simulink model "shield_test_model"  (R2024b)
settings: Solver=FixedStepDiscrete  StartTime=0.0  StopTime=5  FixedStep=1  RelTol=1e-3
libraries: simulink x1
settings Model: Creator=luiz-villa  LastModifiedBy=luiz-villa

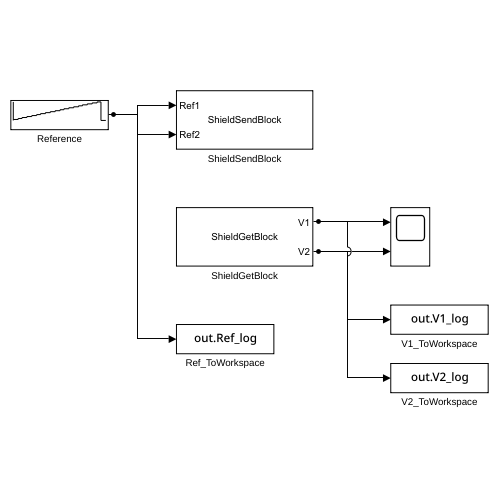
[thumbnail: Simulink's stored preview of the top-level diagram]
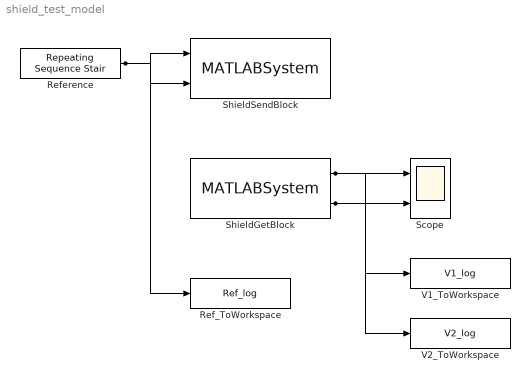
== system shield_test_model ==
  Ref_ToWorkspace : ToWorkspace  VariableName=Ref_log  SampleTime=-1
  Reference : simulink/Sources/Repeating Sequence Stair  OutValues=[5.5 6 6.5 7 7.5 8 8.5 9 9.5 10 10.5 11 11.5 12 12.5 13 13.5 14 14.5 5]  tsamp=1  OutMin=[]  OutMax=[]  OutDataTypeStr=double  OutputDataTypeScalingMode=double  OutDataType=fixdt(0,8)  ConRadixGroup=Best Precision: Vector-wise  OutScaling=2^-12
  Scope : Scope  NumInputPorts=2
  ShieldGetBlock : MATLABSystem  System=ShieldGetBlock  SampleTime=1  VendorID=2fe3  ProductID=0101  Interactive=off
      mask Type: ShieldGetBlock
      mask Display:
      | disp('ShieldGetBlock');
      | port_label('output',1,'V1');
      | port_label('output',2,'V2');
  ShieldSendBlock : MATLABSystem  System=ShieldSendBlock  SampleTime=1  VendorID=2fe3  ProductID=0101  Interactive=off
      mask Type: ShieldSendBlock
      mask Display:
      | disp('ShieldSendBlock');
      | port_label('input',1,'Ref1');
      | port_label('input',2,'Ref2');
  V1_ToWorkspace : ToWorkspace  VariableName=V1_log  SampleTime=-1
  V2_ToWorkspace : ToWorkspace  VariableName=V2_log  SampleTime=-1
  wires:
  Reference/1 -> ShieldSendBlock/1, ShieldSendBlock/2, Ref_ToWorkspace/1
  ShieldGetBlock/1 -> Scope/1, V1_ToWorkspace/1
  ShieldGetBlock/2 -> Scope/2, V2_ToWorkspace/1
